simulink model "model_z_opazovalnikom"  (R2022a)
settings: Solver=ode45  StartTime=0.0  StopTime=20  RelTol=1e-3  EnableMultiTasking=on
values from neighbouring files (symbols this model uses):
  A = [ 0.8, 1;-.4, 0]    [SS_ParamState_Ao_RLS_ex1.m]    (also in untitled.m = model_PS.A)
  avg_dT = sum_dT/N    (= 0)    [untitled.m]
  B = model_PS.B    [untitled.m]
  C = model_PS.C    [untitled.m]
  D = model_PS.D    [untitled.m]
  K = place(a,b,[-0.394764, -0.418224])    [observer_without_feedback_systems.m]    (also in untitled.m = model_PS.K)
  L = P*varphi/(FF + varphi'*P*varphi)    [SS_ParamState_Ao_RLS_ex1.m]    (also in observer_without_feedback_systems.m = L_anastrofos'; untitled.m = L_T')
libraries: cstblocks x1
settings Model: Creator=Lazaros  LastModifiedBy=EonZ
settings SolverCC: AlgebraicLoopSolver=TrustRegion
settings DataIOCC: LimitDataPoints=on  SaveFormat=Array  ReturnWorkspaceOutputs=off
settings OptimizationCC: LifeSpan=inf
settings DebuggingCC: UnderspecifiedInitializationDetection=Classic  MergeDetectMultiDrivingBlocksExec=none  SolverPrmCheckMsg=warning  UnconnectedInputMsg=warning  UnconnectedOutputMsg=warning  UnconnectedLineMsg=warning  StateNameClashWarn=warning  SFUnexpectedBacktrackingDiag=warning  SFNoUnconditionalDefaultTransitionDiag=warning  SFExecutionAtInitializationDiag=none  SFMachineParentedDataDiag=warning  ArithmeticOperatorsInVariantConditions=warning
settings HardwareCC: ProdBitPerPointer=32  ProdBitPerSizeT=32  ProdBitPerPtrDiffT=32  ProdLargestAtomicFloat=None  ProdIntDivRoundTo=Undefined  ProdEndianess=Unspecified  ProdWordSize=32  ProdHWDeviceType=32-bit Generic
settings ModelReferenceCC: PropagateSignalLabelsOutOfModel=off
settings SFSimCC: SimUseLocalCustomCode=off  CustomCodeUndefinedFunction=UseInterfaceOnly
settings RTWCC: RTWUseLocalCustomCode=off  DLArmComputeVersion=19.05
settings CodeAppCC: StateflowObjectComments=on
settings GRTTargetCC: TargetLangStandard=C89/C90 (ANSI)
settings ConfigComp: CovMetricSettings=dw  CovSaveCumulativeToWorkspaceVar=on  CovSaveSingleToWorkspaceVar=on  CovExternalEMLEnable=off

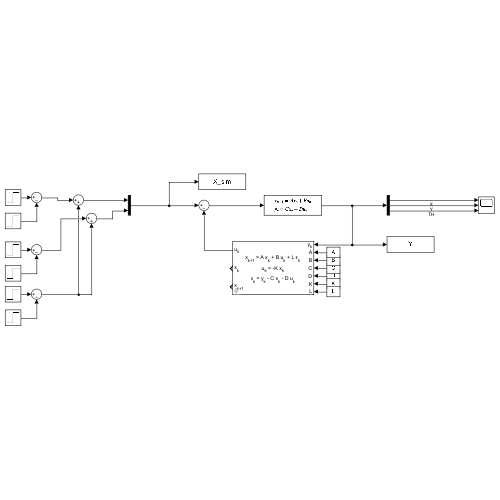
[thumbnail: Simulink's stored preview of the top-level diagram]
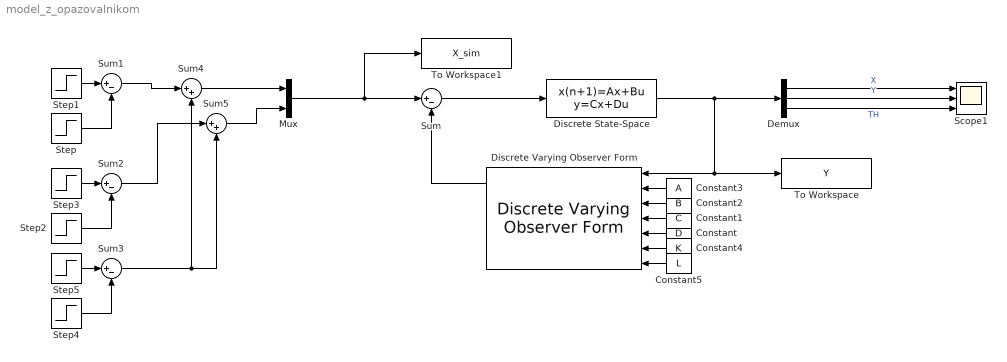
== system model_z_opazovalnikom ==
  Constant : Constant  Value=D
  Constant1 : Constant  Value=C
  Constant2 : Constant  Value=B
  Constant3 : Constant  Value=A
  Constant4 : Constant  Value=K
  Constant5 : Constant  Value=L
  Demux : Demux  Outputs=3
  Discrete State-Space : DiscreteStateSpace  A=A  B=B  C=C  D=D  SampleTime=avg_dT
  Discrete Varying Observer Form : cstblocks/Linear Parameter Varying/Discrete Varying Observer Form  x0=0  Ts=avg_dT  OutputX=on  OutputDX=on
      settings: SourceProductBaseCode=CT
  Mux : Mux  Inputs=2
  Scope1 : Scope  NumInputPorts=3
  Step : Step  Time=5  After=1500  SampleTime=0
  Step1 : Step  Time=0  After=1500  SampleTime=0
  Step2 : Step  Time=11  After=1500  SampleTime=0
  Step3 : Step  Time=6  After=1500  SampleTime=0
  Step4 : Step  Time=17  After=1500  SampleTime=0
  Step5 : Step  Time=12  After=1500  SampleTime=0
  Sum{,1..3} (4 alike) : Sum  Inputs=|+-
  Sum4 : Sum  Inputs=|++
  Sum5 : Sum  Inputs=|++
  To Workspace : ToWorkspace  VariableName=Y  SaveFormat=Structure With Time  SampleTime=-1
  To Workspace1 : ToWorkspace  VariableName=X_sim  SaveFormat=Structure With Time  SampleTime=-1
  wires:
  Demux/1 -> Scope1/1  "X"
  Demux/2 -> Scope1/2  "Y"
  Demux/3 -> Scope1/3  "TH"
  Discrete State-Space/1 -> Demux/1, Discrete Varying Observer Form/1, To Workspace/1
  Constant/1 -> Discrete Varying Observer Form/5
  Sum/1 -> Discrete State-Space/1
  Discrete Varying Observer Form/1 -> Sum/2
  Constant1/1 -> Discrete Varying Observer Form/4
  Constant2/1 -> Discrete Varying Observer Form/3
  Constant3/1 -> Discrete Varying Observer Form/2
  Constant4/1 -> Discrete Varying Observer Form/6
  Constant5/1 -> Discrete Varying Observer Form/7
  Step1/1 -> Sum1/1
  Step/1 -> Sum1/2
  Step2/1 -> Sum2/2
  Step3/1 -> Sum2/1
  Step5/1 -> Sum3/1
  Step4/1 -> Sum3/2
  Sum4/1 -> Mux/1
  Sum5/1 -> Mux/2
  Sum3/1 -> Sum4/2, Sum5/2
  Sum2/1 -> Sum5/1
  Sum1/1 -> Sum4/1
  Mux/1 -> To Workspace1/1, Sum/1
